simulink model "BallAndPlate"  (R2024a)
settings: Solver=VariableStepAuto  StartTime=0.0  StopTime=inf  FixedStep=0.001  MaxStep=0.01  RelTol=1e-3
PostLoadFcn:
  | % Resize the model window
  | set(0,"Units","pixels")
  | sSize = get(0,"screensize");
  | set_param(gcs,'location',...
  |     [1,sSize(4)*0.01,round(sSize(3)/2),sSize(4)*0.96]);
  | 
  | % Reset the zoom
  | set_param(gcs, 'ZoomFactor','FitSystem')
undefined symbols (not defined in the file): X, Y, Z
libraries: sm_lib x44, fl_lib x30, nesl_utility x7, simulink_extras x2
(part 1 of 3)
settings Model: Creator=Rocksmithed  LastModifiedBy=callie
settings DebuggingCC: UnconnectedInputMsg=warning  UnconnectedOutputMsg=warning  UnconnectedLineMsg=warning
settings ModelReferenceCC: EnableRefExpFcnMdlSchedulingChecks=on
settings RTWCC: GPUComputeCapability=3.5  DLArmComputeVersion=19.05
settings ExplorerConfigSet: InternalSimMechanicsExplorerSettings="<ExplorerConfiguration><canonicalview>default</canonicalview><AnimationSetting><BasePlaybackSpeed>1.0</BasePlaybackSpeed><PlaybackSpeedFactor>1.0</PlaybackSpeedFactor></AnimationSetting><TilePanel><TileInfo><Tiles Columns=\"2\" Count=\"4\" Rows=\"3\"><Column Weight=\"0.5\"/><Column Weight=\"0.5\"/><Row Weight=\"0.2495\"/><Row Weight=\"0.2818\"/><Row Weight=\"0.4688\"/><Tile Height=\"2\" Width=\"1\" X=\"0\" Y=\"0\"/><Tile Height=\"1\" Width=\"1\" X=\"1\" Y=\"0\"/><Tile Height=\"1\" Width=\"1\" X=\"1\" Y=\"1\"/><Tile Height=\"1\" Width=\"2\" X=\"0\" Y=\"2\"/></Tiles></TileInfo><SceneInfo><SceneViewer><BGColor><R>1</R><G>1</G><B>1</B></BGColor><Camera><DoPerspective>off</DoPerspective><Position><X>0.00673320048370945525</X><Y>0.00820886465560413496</Y><Z>0.952842467818886485</Z></Position><Center><X>0.00673320048370945525</X><Y>0.00820886465560413496</Y><Z>-0.0471575321811135151</Z></Center><Up><X>0</X><Y>1</Y><Z>-0</Z></Up><ViewLimDist>1</ViewLimDist><YLim>0.252956806096853504</YLim><XLim>0.164816770941252994</XLim></Camera></SceneViewer><SceneViewer><BGColor><R>1</R><G>1</G><B>1</B></BGColor><Camera><DoPerspective>off</DoPerspective><Position><X>0.000406016682317221749</X><Y>-0.996637357431014559</Y><Z>-0.0310478397834132239</Z></Position><Center><X>0.000406016682317221749</X><Y>0.00336264256898544805</Y><Z>-0.0310478397834132239</Z></Center><Up><X>0</X><Y>-0</Y><Z>1</Z></Up><ViewLimDist>1</ViewLimDist><YLim>0.114000464555284911</YLim><XLim>0.159650001227855692</XLim></Camera></SceneViewer><SceneViewer><BGColor><R>1</R><G>1</G><B>1</B></BGColor><Camera><DoPerspective>off</DoPerspective><Position><X>1.00185081307351975</X><Y>0.000111850688780237417</Y><Z>-0.0209342650449971385</Z></Position><Center><X>0.00185081307351975255</X><Y>0.000111850688780237417</Y><Z>-0.0209342650449971385</Z></Center><Up><X>-0</X><Y>0</Y><Z>1</Z></Up><ViewLimDist>1</ViewLimDist><YLim>0.128805719692334897</YLim><XLim>0.15965000122785572</XLim></Camera></SceneViewer><SceneViewer><BGColor><R>1</R><G>1</G><B>1</B></BGColor><Camera><DoPerspective>off</DoPerspective><Position><X>0.565722614442947691</X><Y>-0.563172639196256042</Y><Z>0.537824528089690168</Z></Position><Center><X>-0.0116276547466781979</X><Y>0.0141776299933697551</Y><Z>-0.0395257410999356046</Z></Center><Up><X>-0.408248290463863073</X><Y>0.408248290463863073</Y><Z>0.816496580927726145</Z></Up><ViewLimDist>1</ViewLimDist><YLim>0.2725303104620449</YLim><XLim>0.40723279189454642</XLim></Camera></SceneViewer></SceneInfo></TilePanel><MechEditorPanel><Cameras><Camera><Id>Camera1</Id><Value><Name>Camera1</Name><NativeCamera><PositionKeyframeSet><Keyframe><Time>10</Time><Value><X>0.25964088459989382</X><Y>-0.28762095410947258</Y><Z>0.082651797281669104</Z></Value></Keyframe></PositionKeyframeSet><CenterKeyframeSet><Keyframe><Time>10</Time><Value><X>0.0055924714532661901</X><Y>0.015756426590547323</Y><Z>-0.1039414113209412</Z></Value></Keyframe></CenterKeyframeSet><UpVectorKeyframeSet><Keyframe><Time>10</Time><Value><X>-0.26891217970240533</X><Y>0.33110613174141906</Y><Z>0.90446391256419689</Z></Value></Keyframe></UpVectorKeyframeSet></NativeCamera></Value></Camera></Cameras><GfxPanelCameraMap/><VideoCreator><PlaybackSpeedRatio>1.0</PlaybackSpeedRatio><FrameRate>30</FrameRate><VideoFormat>Motion JPEG AVI</VideoFormat><FrameSize>auto</FrameSize></VideoCreator></MechEditorPanel></ExplorerConfiguration>"

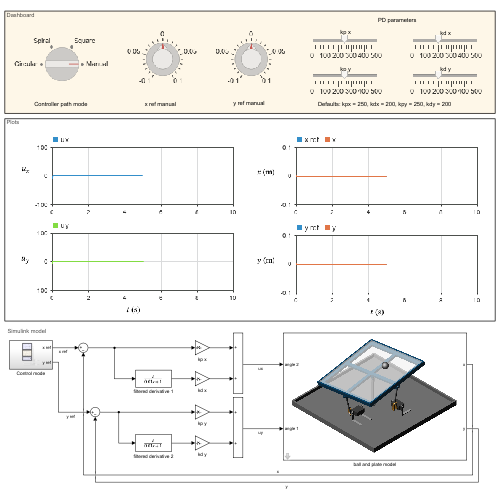
[thumbnail: Simulink's stored preview of the top-level diagram]
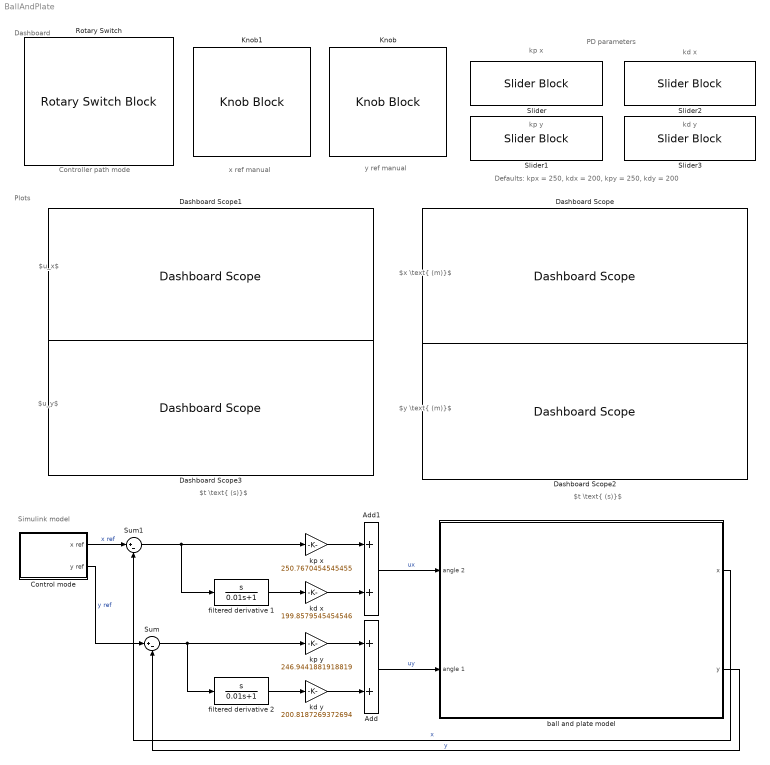
== system BallAndPlate ==
  note: Plots
  note: $u_x$
  note: $t \text{ (s)}$
  note: $x \text{ (m)}$
  note: $t \text{ (s)}$
  note: Simulink model
  note: Dashboard
  note: Controller path mode
  note: $u_y$
  note: $y \text{ (m)}$
  note: x ref manual
  note: y ref manual
  note: kp x
  note: Defaults: kpx = 250, kdx = 200, kpy = 250, kdy = 200
  note: PD parameters
  note: kd x
  note: kp y
  note: kd y
  Add : Sum
  Add1 : Sum
  Control mode : Subsystem
  Dashboard Scope : DashboardScope  TimeSpan=10  Ymin=-0.15  Ymax=0.15  ScaleAtStop=off  UpdateMode=Scroll
  Dashboard Scope1 : DashboardScope  TimeSpan=10  Ymin=-100  Ymax=100  ScaleAtStop=off  UpdateMode=Scroll
  Dashboard Scope2 : DashboardScope  TimeSpan=10  Ymin=-0.15  Ymax=0.15  ScaleAtStop=off  UpdateMode=Scroll
  Dashboard Scope3 : DashboardScope  TimeSpan=10  Ymin=-100  Ymax=100  ScaleAtStop=off  UpdateMode=Scroll
  Knob : KnobBlock  LabelPosition=Hide  ScaleMin=-0.1  ScaleMax=0.1  TickInterval=0.05
  Knob1 : KnobBlock  LabelPosition=Hide  ScaleMin=-0.1  ScaleMax=0.1  TickInterval=0.05
  Rotary Switch : RotarySwitchBlock  LabelPosition=Hide
      settings: Values={{'Circular', 'Spiral', 'Square', 'Manual'}, [0 1 2 3]}
  Slider{,1..3} (4 alike) : SliderBlock  LabelPosition=Hide  ScaleMax=500  TickInterval=100
  Sum : Sum  Inputs=|+-
  Sum1 : Sum  Inputs=|+-
  ball and plate model : Subsystem  mask{mball=1, rball=1}
      mask prompts: mball "Ball mass (kg)"; rball "Ball radius (cm)"
      mask help: Ball and plate model
      mask Display: image('image_0.png');
  filtered derivative 1 : TransferFcn  Numerator=[1 0]  Denominator=[0.01 1]
  filtered derivative 2 : TransferFcn  Numerator=[1 0]  Denominator=[0.01 1]
  kd x : Gain  Gain=199.8579545454546
  kd y : Gain  Gain=200.8187269372694
  kp x : Gain  Gain=250.7670454545455
  kp y : Gain  Gain=246.9441881918819
  wires:
  Sum/1 -> kp y/1, filtered derivative 2/1
  ball and plate model/2(y) -> Sum/2  "y"
  ball and plate model/1(x) -> Sum1/2  "x"
  kp y/1 -> Add/1
  filtered derivative 2/1 -> kd y/1
  kd y/1 -> Add/2
  Add/1 -> ball and plate model/2(angle 1)  "uy"
  kd x/1 -> Add1/2
  Add1/1 -> ball and plate model/1(angle 2)  "ux"
  kp x/1 -> Add1/1
  filtered derivative 1/1 -> kd x/1
  Sum1/1 -> kp x/1, filtered derivative 1/1
  Control mode/1(x ref) -> Sum1/1  "x ref"
  Control mode/2(y ref) -> Sum/1  "y ref"

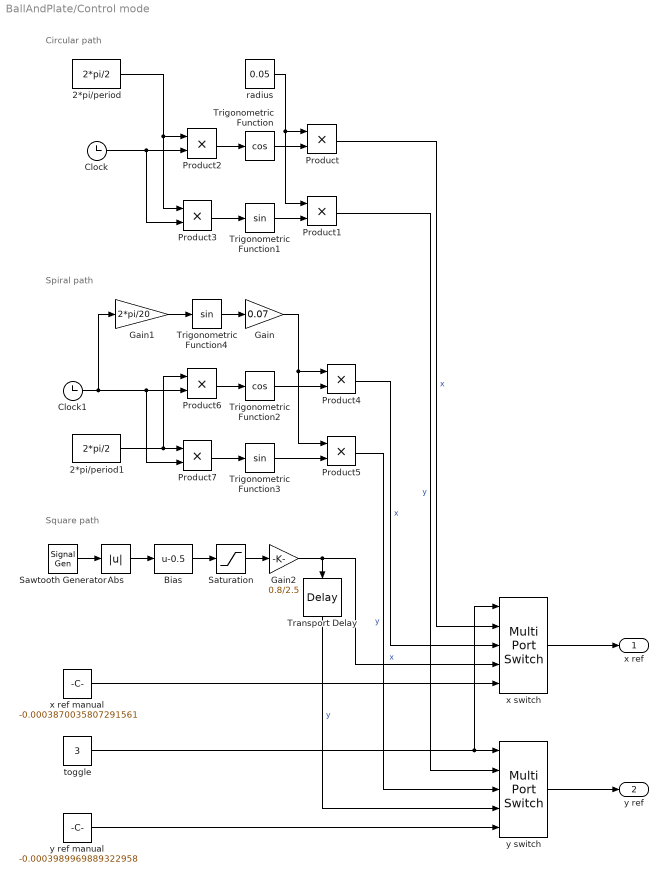
== system BallAndPlate/Control mode ==
  note: Square path
  note: Spiral path
  note: Circular path
  2*pi/period : Constant  Value=2*pi/2
  2*pi/period1 : Constant  Value=2*pi/2
  Abs : Abs  SaturateOnIntegerOverflow=off
  Bias : Bias  Bias=-0.5  SaturateOnIntegerOverflow=off
  Clock : Clock
  Clock1 : Clock
  Gain : Gain  Gain=0.07
  Gain1 : Gain  Gain=2*pi/20
  Gain2 : Gain  Gain=0.8/2.5
  Product{,1..7} (8 alike) : Product
  Saturation : Saturate  UpperLimit=0.25  LowerLimit=-0.25
  Sawtooth Generator : SignalGenerator  WaveForm=sawtooth  Frequency=0.05
  Transport Delay : TransportDelay  DelayTime=5  BufferSize=10000
  Trigonometric Function : Trigonometry  Operator=cos
  Trigonometric Function1 : Trigonometry
  Trigonometric Function2 : Trigonometry  Operator=cos
  Trigonometric Function3 : Trigonometry
  Trigonometric Function4 : Trigonometry
  radius : Constant  Value=0.05
  toggle : Constant  Value=3
  x ref manual : Constant  Value=-0.0003870035807291561
  x switch : MultiPortSwitch  DataPortOrder=Zero-based contiguous  Inputs=4  zeroidx=on  SaturateOnIntegerOverflow=off  InputSameDT=off
  y ref manual : Constant  Value=-0.0003989969889322958
  y switch : MultiPortSwitch  DataPortOrder=Zero-based contiguous  Inputs=4  zeroidx=on  SaturateOnIntegerOverflow=off  InputSameDT=off
  x ref : Outport
  y ref : Outport  Port=2
  wires:
  x switch/1 -> x ref/1
  y switch/1 -> y ref/1
  Gain1/1 -> Trigonometric Function4/1
  Gain/1 -> Product4/1, Product5/1
  Trigonometric Function4/1 -> Gain/1
  Trigonometric Function3/1 -> Product5/2
  2*pi/period1/1 -> Product6/1, Product7/1
  Product7/1 -> Trigonometric Function3/1
  Clock1/1 -> Product6/2, Product7/2, Gain1/1
  Product4/1 -> x switch/3  "x"
  Product5/1 -> y switch/3  "y"
  Trigonometric Function2/1 -> Product4/2
  Product6/1 -> Trigonometric Function2/1
  Product1/1 -> y switch/2  "y"
  y ref manual/1 -> y switch/5
  x ref manual/1 -> x switch/5
  Clock/1 -> Product3/2, Product2/2
  Product3/1 -> Trigonometric Function1/1
  2*pi/period/1 -> Product3/1, Product2/1
  Product2/1 -> Trigonometric Function/1
  Trigonometric Function1/1 -> Product1/2
  Trigonometric Function/1 -> Product/2
  radius/1 -> Product/1, Product1/1
  Product/1 -> x switch/2  "x"
  toggle/1 -> x switch/1, y switch/1
  Saturation/1 -> Gain2/1
  Sawtooth Generator/1 -> Abs/1
  Gain2/1 -> x switch/4, Transport Delay/1  "x"
  Abs/1 -> Bias/1
  Bias/1 -> Saturation/1
  Transport Delay/1 -> y switch/4  "y"
